simulink model "CM13_2024a_MachE_for_UA_HIL"  (R2024a)
settings: Solver=ode1  StartTime=0.0  StopTime=Inf  FixedStep=0.001  RelTol=1e-3  EnableMultiTasking=on
PreLoadFcn:
  | % if ~length(which('cmcmd')), cmenv; end
PostLoadFcn:
  | if any(exist('dsrtsu_mdlpostloadfcn', 'file') ~= 0), dsrtsu_mdlpostloadfcn('Execute', bdroot); end
InitFcn:
  | , if any(exist('rtifpga_mdlclblib', 'file') ~= 0), rtifpga_mdlclblib('Init', bdroot); end,
  | , if any(exist('dsmpb_private', 'file') ~= 0), dsmpb_private('dsmpb_mdlclblib', 'Init', bdroot); end,
values from neighbouring files (symbols this model uses):
  CoastDown =     [Run_Simulink.mat]
  limitedMCT =     [Run_Simulink.mat]
  MCT =     [Run_Simulink.mat]
  pMCT =     [Run_Simulink.mat]
  RealSimPara =     [Run_Simulink.mat]
  Ref_speed = [13 13.007895099 13.015778396 13.023649891 13.031509584 13.039357475 13.047193564 13.055017851 13.062830336 13.070631019 13.0784199 13.086196979 ... (2669 elements, 2669x1)]    [Ref_speed_and_time.mat]
  Ref_time = [0 0.01 0.02 0.03 0.04 0.05 0.06 0.07 0.08 0.09 0.1 0.11 ... (2669 elements, 2669x1)]    [Ref_speed_and_time.mat]
  US06 =     [Run_Simulink.mat]
undefined symbols (not defined in the file or in its folder): AccelCmd, ActTqLF_Nm_, ActTqLR_Nm_, ActTqRF_Nm_, ActTqRR_Nm_, BattChargeLimitMaxPwr, BattChargeLimitSocBpts, BattChargeLimitTbl, BattChrgCapcty, BattDischargeLimitSocBpts, BattDischargeLimitTbl, BattDischargeMaxPwr, BattNumCellsParallel, BattNumCellsSeries, BattOpenVoltCapBpts, BattOpenVoltTbl, BattResistSocBpts, BattResistTbl, BattResistTempBpts, BrakeMaxPrs, BrakeMaxTrq, ChassisDistCg2FrontAxle, ChassisDistCg2RearAxle, ChassisVehMass, CltchCmd, DecelCmd, DiffRatio, DiscIntNeverNeededParam, EnvGravCnst, EnvPrs, EnvTemp, FuelSpecificGrav, GearCmd, h, InitStates, lgSw, MtrEffSpdBpts, MtrEffTbl, MtrEffTrqBpts, MtrPwrMax, MtrTrqMax, planned_speed, planned_time, ref_speed, ref_time, rticanmm_blockfcn, rticanmm_initfcn, SteeringCmd, SupvsryCtrlRegenBrkCutOffTbl, SupvsryCtrlRegenSpdBpts, TestScnrioCycleNum, VEH
libraries: simulink x264, VSIGenLib x262, etargetslib x201, dsmpblib x161, CarMaker4SL x142, rtimmsu_dsrtlib x32, vehdynlibtire x24, autolibshared x19, vehdynlibsuspension x14, vehdynlibtirecommon x14, autolibutils x10, VsrLibWheel x8
(part 1 of 48)
PreSaveFcn:
  | , if any(exist('dsmpb_private', 'file') ~= 0), dsmpb_private('dsmpb_mdlclblib', 'PreSave', bdroot); end,
CloseFcn:
  | , if any(exist('dsmpb_private', 'file') ~= 0), dsmpb_private('dsmpb_mdlclblib', 'Close', bdroot); end,
settings Model: DataDictionary=DdPassengerEv.sldd  DSMPB_ID_DATA={'10310',struct('BlockId','12f36d3f-3469-493d-9061-ec8dccf8ad98','SignalIds',{{'1d9f63b3-fb1e-42b1-b986-118c3f8e1a5c'}}),'10386',struct('BlockId','00ced8af-8f81-4d96-bdd5-55bcf75b326f','SignalIds',{{'de137f90-4176-4482-a330-2263656912b8','2543f34f-34c7-418b-b364-51a674ed6701','2ea953f6-258f-43af-80b9-296d510766cd','e026f27b-656f-438f-b55c-47d82fb791c0','910672e4-b9cf-495b-ab37-fd8fda6aed4f'}}),'12703',struct('BlockId','d5c239de-9c28-471f-8378-f6be1ca07354','SignalIds',{{'0523bd6f-493f-4b67-9a37-7f171dccadcf'}}),'12768',struct('BlockId','6f08745e-850f-4fc7-99c6-1c2500a944b6','SignalIds',{{'dd9ed340-905e-44be-a84a-808b15caceaf'}}),'12769',struct('BlockId','22e84ecd-9087-47b3-b69e-68ef51f81dd7','SignalIds',{{'a20bbc9a-e0b1-414e-ad46-369f23f85a67'}}),'12770',struct('BlockId','ea678779-fea7-480d-bd70-6fd84e893b88','SignalIds',{{'514a1219-de9e-4b45-a8c1-f0eec9473038'}}),'12849',struct('BlockId','8d70948c-1b65-454e-80b6-488007125876','SignalIds',{{'85315227-9b7c-473a-8f8a-5b34e6a28267'}}),'12850',struct('BlockId','4f95301f-61bc-40f6-b577-b49e4cb81cdc','SignalIds',{{'72592b21-14ea-414f-bad7-eb7b114d5a0e'}}),'12851',struct('BlockId','ac6bf72f-e1b6-495e-9e4b-894c6746d1a0','SignalIds',{{'f9b0dee9-4290-4449-a8ea-24130731cef7'}}),'12857',struct('BlockId','6b10a409-0c93-4934-ac05-3e71bd8b4d56','SignalIds',{{'a7480ea2-3795-4920-80c4-197fbf749da8'}}),'12858',struct('BlockId','c572fa2b-15ad-41aa-81fe-e8bbbed5f461','SignalIds',{{'06004834-c0b9-4189-81f2-9fc7072798a8'}}),'12859',struct('BlockId','1c6655ba-19a9-4cd0-926e-198f5e98e044','SignalIds',{{'527b24a8-f319-412d-b942-e50c619d5c98'}}),'12892',struct('BlockId','cdf75210-031f-4acf-a586-f109f3081db8','SignalIds',{{'0eebc661-386c-4153-975b-200fc7917c9c'}}),'12893',struct('BlockId','bbaf36c3-78c2-4f66-b911-8060317349d0','SignalIds',{{'d6526e73-4ca6-4a7b-95d2-0da9f3f3bb3c'}}),'13389',struct('BlockId','e0063ee2-603a-42f4-80ca-58f4b3e23b5a','SignalIds',{{'5991410c-cc0f-42d8-93ab-94a3aee0e461'}}),'13397',struct('BlockId','0909c5b7-dd88-48d1-abaf-d3324e1e7649','SignalIds',{{'4919af6e-e187-49a8-a288-eb81d671cc8d','e79f3ee3-b422-4636-bed9-529d41626698','8262c110-cc1a-4ba5-8eaa-8176657d5cc1','37cd9612-221b-4281-99cc-4b4394a20fc4','891ab062-363b-41ce-bada-c2e12e4ea74e','cee21b9f-e160-4a13-ad59-480745ef8104','5f399649-cfff-40b7-aace-1cbf0d264993','83711fe8-b2d9-45eb-9dbc-3c51b17f7674','cb7a5443-6e0a-467a-bec9-cb544ca1c2f3'}}),'13398',struct('BlockId','6c3e85bd-363e-417f-8d2b-de29daccd343','SignalIds',{{'573cb497-90a4-454c-b538-934bab3fb65f','4def0a6e-14a7-45d5-ac89-6368950213ca','1faf2666-945f-46a8-b93d-c749f0ec4d9a','255bf974-2f16-4189-ac8d-0135b7b658d1','48de1ef3-4aa0-4b6a-a60f-af052b360edb','b8858909-8a89-4d3a-b884-12439f2c8ddf','7a91e7da-847c-4fed-ac2b-a72166cf88c2','47f03b93-48b4-4b1e-998e-43cb7f69ff32','20de7b31-4a1c-4f17-8b36-e3a815e77dd8'}}),'13399',struct('BlockId','85425dac-ee7a-4bf9-975b-095d7c4dcb51','SignalIds',{{'31f78e19-b7be-40a1-8403-a05f60a9fdd4','54ddbf4f-4a1f-42da-9a57-0479aebd4948','43029009-e5b6-4870-adc7-930fcda97230','fa37dcdd-61b9-427c-8689-e42eb565dcdf','b21329b6-313d-4a80-bafb-48f151b485d6','5e1f092d-d023-45af-8e83-81d7db73fe71','575eb17a-767f-476b-b29e-c7c824fb5c3f'}}),'13400',struct('BlockId','6d25d758-e342-4d0e-a1c0-e299c4d680c4','SignalIds',{{'e44851b8-4536-4fec-815f-e58aadf79b08','786f882c-9ff4-429e-a7c6-066a4a17b40d','45a0b4ca-80fc-40f6-b1e6-27e5d7b713ae','92135807-4645-4e98-a81c-4de8955bda43'}}),'13401',struct('BlockId','9d879170-0616-4207-b220-fd282f7b9eac','SignalIds',{{'ac11617f-dbda-443f-993c-c6fbbd6ab47f','34ee468f-8712-4e56-b2fa-57cfaf4d46a9','6645cccf-1e45-43d8-b9ae-20ca198c39ab','cb498cb6-3450-42a8-8043-9ca37324ef60'}}),'13419',struct('BlockId','43998d1e-e7ec-4013-910a-1b0f7c017215','SignalIds',{{'8d4301fb-cf57-464e-a726-f69194925ee2','74880e10-5ea6-4fdb-851a-33803dc7f46b','6c464908-c4ce-42ec-bd75-49943b5eafb2'}}),'13420',struct('BlockId','e0c48fa1-6a1e-4e4d-a91e-2ca8abf999f7','SignalIds',{{'607599af-e337-41d8-9854-a4c9e0dad2db'}}),'13596',struct('BlockId','2654cd16-1152-433b-ac1a-0269a27feef5','SignalIds',{{'f18cf10c-063a-4024-9056-7b6eead01ef8'}}),'13597',struct('BlockId','4fbf4d76-c906-4f09-a2a6-3f44242523b1','SignalIds',{{'ca8c2ef4-b7df-4c3e-96eb-badff8bb811e'}}),'13598',struct('BlockId','64454236-9a5a-47cb-bb03-f5232c93f512','SignalIds',{{'8d05b93c-46cb-4582-bdb0-e3eb534cd12f'}}),'13599',struct('BlockId','56f11289-4ff5-403f-9839-a82d5b54af48','SignalIds',{{'701aa950-68b2-4ec2-a6c8-d52ba2bcd249'}}),'13600',struct('BlockId','1b0cbb7a-7a69-42f5-9c01-3c170bbe0689','SignalIds',{{'b4817d5e-c060-44db-b5d8-db08f2e889fe'}}),'13601',struct('BlockId','d433aed8-57c8-49ee-bc14-5afa6b45083e','SignalIds',{{'b98e298f-f0b2-450f-b551-4d44ae548aeb'}}),'13602',struct('BlockId','74c1e029-d9b4-4c74-ba04-02cb146b3796','SignalIds',{{'2376ff9a-21ba-487c-823a-f7ab79b5155e'}}),'13603',struct('BlockId','b93cc2c6-1b2f-4cdd-9704-427da45e27fa','SignalIds',{{'e0dbe44a-cc69-4581-af9e-328a90ef1812'}}),'13658',struct('BlockId','9b6a6234-f391-402b-b330-759f0b2f72d0','SignalIds',{{'f5fe7a89-d43d-45da-86dd-9843ffe74786','2b32734c-d92c-4dda-80af-1b7131aac85a','66759741-14ac-464f-974d-6dad41e59beb','2edbc071-bd43-46c5-b834-94c1dd327098','9c492387-aa58-4280-9aa7-95e0d8fe3f01'}}),'13705',struct('BlockId','68defd7b-f812-4d52-8a6f-ab6878e61943','SignalIds',{{'4f92870f-0cc2-427d-ae47-c99b1dd6cbba','06b4d400-fc57-44d8-a8bf-2ee416fb1012','3c4d588d-1906-4006-895e-8fe51fefc384','17ee284c-01e4-44e1-bb0a-5d8f70a5896a','26334ad1-9d74-4531-8fa5-fc841244f7b7'}}),'13706',struct('BlockId','a130b25d-d8e8-4208-976d-a8c4ca165afd','SignalIds',{{'552f6f50-3547-418f-870a-1f967936f110','0b37453a-0fe5-4ef2-9e52-b923bd5f02d1'}}),'13708',struct('BlockId','00e457ba-09c7-460a-8fa7-b07e79c909cf','SignalIds',{{'e82db465-0dc5-4428-9d60-01905a71cf23','4ec6b1dd-22b3-4774-a6d4-013670478f6c','0cfd2b7c-eff3-4a40-9c90-09f8ecc43c65','7fb521d2-5b57-4a71-a2ea-6ccd095d0c8d','0190859d-2e3e-4484-8825-99cc894eeb49','d42c3cfc-c223-4053-93a1-8afdb70193a2'}}),'13709',struct('BlockId','8d7eeffa-57e3-4b4f-84b4-4cf68f00cd15','SignalIds',{{'88d51ca8-c776-4b07-b10b-ccd6deed6120','a40c7935-a03c-429a-b8e5-73a50a866f27','336de083-ceaa-4113-b8ce-44c9d005ade5'}}),'13855',struct('BlockId','35cad703-acce-4db5-b1e1-ecf2bb4e8a68','SignalIds',{{'2413f319-8556-4695-8444-c4a35b6cf84b'}}),'13860',struct('BlockId','2eebd351-5d35-4dc4-8238-5f7ff35a1c0f','SignalIds',{{'a476340e-b09d-48f6-95b7-2a6d936a9864'}}),'13862',struct('BlockId','4cef6eab-d55f-4319-80e1-8f29e1b6ca28','SignalIds',{{'2e3a24d0-c0d4-45f2-b3c3-1f40fcbb9025'}}),'14002',struct('BlockId','b7b542e5-4f26-43e0-af00-0765c47a7be4','SignalIds',{{'b43777bc-78e7-420d-b9c7-924ec3bc0020','d77c6156-a416-4862-952d-fd0c5f3a4268','166ad4cd-0ca0-426d-ae27-28c6d47f4290','eab723f9-c9cb-4bd9-ad26-d5cc16da50d8','51d6cafe-d61a-4ece-aa88-83317d4387c0'}}),'14003',struct('BlockId','690bdae9-44d4-406d-99dc-0fe1eca8290a','SignalIds',{{'6c80bdc4-ebd8-45a9-864d-b0c96184911a','403fc45c-435b-48b1-828c-9b32406d4289'}}),'14004',struct('BlockId','13d1cad0-5e25-434f-942f-03b54b407f13','SignalIds',{{'b6797402-dc17-4702-af16-93cfc7bfd2c6'}}),'14017',struct('BlockId','3f4708ba-c9ff-47b1-b444-ebd911931fcd','SignalIds',{{'60f0e601-d4a2-413a-9877-bf51a75436d8','e9d10586-6241-4149-aed5-74580bd4b32f'}}),'14484',struct('BlockId','7a1b6b1f-e57f-4ef6-b9b6-c00e3a7c18b3','SignalIds',{{'c517a655-c3ae-4248-84d8-a509b79721e3'}}),'14560',struct('BlockId','4b6a7fa7-390d-4c9d-8eb2-f646fefb0631','SignalIds',{{'fda74313-f654-4561-8d6e-e1fa65ef5a21','7ffdead9-2939-42b4-83d3-0e6b32034344','3ef057b8-b6cd-4be8-aee9-398cd49c464f','b4dbcd46-e281-4bb0-843c-cd41170e779c','23ad03d5-e7b7-4ede-a329-18094eaa1732'}}),'14675',struct('BlockId','80315e53-3825-452f-8418-928ce0a5b884','SignalIds',{{'d205fa42-dbb1-4ac4-89fc-174df3da1ad3','8ace96e5-9ccd-4bb6-b3ad-795b8a7818d7'}}),'14676',struct('BlockId','c2ff3260-6d21-42bd-9c67-af339cb9da94','SignalIds',{{'cb4212e4-9c41-4702-928f-e6f7011d53eb','a2441cfe-efec-4f72-80a9-ff18d8aeaeb2'}}),'14677',struct('BlockId','5c259738-61c1-4940-b8c6-678009d700b4','SignalIds',{{'3eaa4d46-076b-4376-8fff-6799fc59ae2c'}}),'14678',struct('BlockId','2b7fdaf0-3bca-4cf8-a01f-16a5ffc40654','SignalIds',{{'7e7316db-c453-4c12-b989-f13ac322e4cc','3324bf27-85f1-4009-b151-35eff7706011'}}),'14748',struct('BlockId','af115fdf-462b-4d46-b5ae-ed48f32a80ce','SignalIds',{{'a2fc24b4-9495-448c-9d68-ee1fbf037ff0','a32c49c5-1f60-4290-a235-9c5ab953ac1f','fbd442c5-8d0d-402d-8b0e-47648da22c93','0dcdade1-2f6f-46b2-a175-bd0a95998b17','aa75d810-8c00-47ac-838d-94ccc8794fde'}}),'14749',struct('BlockId','5bef166d-4a50-45b6-bcd8-c40106e5818d','SignalIds',{{'f4d1b59c-cbd2-4fb4-aba8-393dcc75f58c','0b8133cd-cc0b-4ae3-902f-0805f41a78a0','50798339-b4d9-4001-9b38-71cae5aae466','652cb478-e44a-4f29-9fdc-11278afe8acd','6db05899-163c-4272-b68d-3f23fdc3c2f4'}}),'14863',struct('BlockId','4bdde38d-9bde-4f01-846b-8d6f64c11475','SignalIds',{{'13759f7c-dc26-41c0-a673-d7e6ba4117c6'}}),'14890',struct('BlockId','000dd422-5c9e-49e2-8ae1-d8578451c04f','SignalIds',{{'dd524eb7-1453-448b-a121-3fbe1baeb907','19b407c4-6367-4a79-849c-0e74e550025c','d7d7cf32-1390-4596-8ad8-a7aa1ee97e47','ec108f91-b7ef-4da9-af1a-6887c10d8753'}}),'14895',struct('BlockId','e0a324a1-9c85-4c4d-9120-42a0e22c223f','SignalIds',{{'b3d2bbe9-e87c-45ea-bcce-28bf589283a0','cc171703-e72c-488f-98b6-b3675eb74135','f695ec14-797c-4600-923d-3f8ecde3a7b7'}}),'14908',struct('BlockId','2adb24e4-0efe-45b2-9f22-8475825d43f7','SignalIds',{{'3ceca581-e09a-490b-858b-383b4ff560e2','8daa67bb-bba5-42a9-9ff7-1f642b97bd96'}}),'14916',struct('BlockId','65eb0149-4723-49de-a5d3-69f9fc2610cc','SignalIds',{{'f164dca4-ea5e-462e-b4f1-9f1df6910adb','193413f2-adb8-4371-a123-e7aee3d7ab7f'}}),'15031',struct('BlockId','1f1e6500-410f-49b1-8066-fea9c1ff0cda','SignalIds',{{'ec87fc4e-5b14-4747-9c72-d1e77db60252'}}),'15032',struct('BlockId','6c14e7ad-b236-4cbc-987f-2777f585868c','SignalIds',{{'907d72f5-7c34-4dc8-b661-c51071fe02dc'}}),'15033',struct('BlockId','a2c50340-e125-491b-b6fe-9bd004392e2b','SignalIds',{{'99772446-b668-4d45-9a17-77a327a28077','34fc074f-911c-415d-abca-7890622cc05f'}}),'15034',struct('BlockId','f40daa0e-2494-4582-b47b-fa6e80cc9a9b','SignalIds',{{'904ebebf-fd02-4665-ad45-ede3e402e544','9437c417-61c8-4fd3-8798-da1d3fa95319','fd5d1af9-42ef-4ee3-b09d-926de420ed93','548a470a-bf47-498a-a60e-e5e352f2143e'}}),'15035',struct('BlockId','f52398c5-79fc-42b0-a409-ec3938884e6a','SignalIds',{{'b30d349e-d6a0-44e0-a327-584adaaa49d9'}}),'15036',struct('BlockId','52a4dbb2-6d8c-462d-96a6-dfd44641d89f','SignalIds',{{'289d42f8-ed6e-4801-97a2-d0bf259ebab1','691872a8-7380-4677-9e6c-faf9246f9b43','e0932303-f76d-4dd2-85bc-028033373e8c'}}),'15037',struct('BlockId','0e0291c9-35a5-4563-a570-cb376424caa3','SignalIds',{{'b066e553-674a-4235-9b1a-1f56165c7d67'}}),'2270',struct('BlockId','3bd45aea-114e-4e0b-8274-661c86aceb33','SignalIds',{{'c8b7fc0a-a8e0-4d2f-8a1a-d6be83cb4224'}}),'2773',struct('BlockId','2aba53d9-4d19-4b4d-8397-819e1325edd4','SignalIds',{{'5b2c7b7e-348d-491d-bca0-371c7d75daf6'}}),'2849',struct('BlockId','f460e1ab-e71c-4464-aa19-00052b52454f','SignalIds',{{'30b32590-3625-4bb9-ae32-15e6284ff4a4','66da3457-bf16-43a8-8d28-731e6b8caf4a','952c0afe-8835-4b70-b79b-fdafd7d110e9','fc1acb7d-e31a-4377-87b6-ab40ebaf385e','ba74fcbd-4265-4b9a-9e5b-7274eedbbc92'}}),'3443',struct('BlockId','bf4848e9-a005-4ea5-822a-546d14facefb','SignalIds',{{'59813826-0850-4d64-8d90-ce02e5c4772d'}}),'3444',struct('BlockId','661dc0ac-bd0b-40f3-8260-966d3389d24d','SignalIds',{{'5bd69b46-b717-4764-8a4c-31062ca41d6c'}}),'3445',struct('BlockId','1e60593e-fb4e-4ad7-b476-f227a587c97e','SignalIds',{{'46a8325f-67fa-40bb-92c0-5fbd7b9fd8c0'}}),'3446',struct('BlockId','cf726b69-21f9-4634-b1ea-2afedf885ef4','SignalIds',{{'43cd743a-0c41-42be-aa5c-12364b2a34b1'}}),'3447',struct('BlockId','825c9d59-301a-41c7-ad59-05beda97f4c0','SignalIds',{{'1e421ba1-785f-4677-bc54-4b32ccffbda9'}}),'3448',struct('BlockId','6d4532c8-7821-4780-900f-08e025780dbb','SignalIds',{{'fd5bdd2e-ab61-412d-8d45-c0b4d87df8e1'}}),'3449',struct('BlockId','41cc231b-b267-49ab-a469-ecc9f97ba82b','SignalIds',{{'518b8c22-f5d9-42d6-b2fb-633612b3457c'}}),'3450',struct('BlockId','06ddf642-c8ec-424a-a257-45d7d14fbc9c','SignalIds',{{'191bc148-b179-491d-9c31-5c50bd08bc6c'}}),'3570',struct('BlockId','b840981a-3739-4217-ad3e-20af8bf4bb2c','SignalIds',{{'85ff8f48-ed7c-4597-8ae2-1f0d11eaa759'}}),'3571',struct('BlockId','b44c9645-0f3c-4062-b7ea-542130e6b9d2','SignalIds',{{'0ce735d0-6ea1-4243-b07a-fb60e0271719'}}),'3572',struct('BlockId','a8420ce8-9668-411f-94bd-e6da040620a4','SignalIds',{{'a2d69c3d-b01f-4b76-ba89-e2cf06da7db2'}}),'3648',struct('BlockId','0f5c264c-ffce-4912-adaa-a76aa10f5c95','SignalIds',{{'97ac99fa-5070-4e14-b3c4-316cb4960b65'}}),'3649',struct('BlockId','96f45e98-66f7-475c-982f-1d996f097844','SignalIds',{{'c9d1fa6d-224f-4782-b6fa-e02890b2d4d6'}}),'3650',struct('BlockId','e6f5ddfe-bc8f-44ab-9711-b56df51aee9e','SignalIds',{{'152cb444-4e9c-4a5a-a35b-04356aab4aa1'}}),'3656',struct('BlockId','548c7893-6eac-4873-a730-0dbe400694d8','SignalIds',{{'aed0196a-9e2d-4895-aa85-c8c81f784756'}}),'3657',struct('BlockId','6b692eed-3617-4adc-a523-e5d1ef66fefe','SignalIds',{{'92296544-a098-415a-aa5f-75c942b4cbed'}}),'3658',struct('BlockId','c3916ff6-39b4-422e-aac1-4d4a7e0af62c','SignalIds',{{'7d662d18-9ff5-4e89-b916-88d69295e188'}}),'3738',struct('BlockId','24c81f19-ed3f-4f43-8e7c-e6489392a6df','SignalIds',{{'de091b36-0771-4057-8def-13bdc4ea5265'}}),'3765',struct('BlockId','c267f4c0-5dea-4501-b10d-b1f3fd1bab70','SignalIds',{{'7e394da2-e75e-4490-9c5d-1822b2e5143e','352f2db2-e378-493b-85fb-2e8fa202457f','cd8dd211-ea81-4875-aac8-8e2dcb47c3e2','e1626839-2f5e-4e74-892c-ae50640ccd4b'}}),'3770',struct('BlockId','0b92c14b-9c1e-44ed-9fdf-522f83f38d39','SignalIds',{{'a6b988fe-26fc-4e12-b5c8-bec22bcb8ac3','7587cd01-78be-44f3-94ad-d5cdaef89f1f','9098a390-037c-49bf-addd-6abb7a5009cd'}}),'3783',struct('BlockId','0e03ea55-0f88-465a-82f3-07c0c55c23a2','SignalIds',{{'d79cfbf9-3eee-42b7-83fe-5ffa59395bb0','ecb26389-60a7-4388-bcd5-c3d076c7daa5'}}),'3791',struct('BlockId','5511d4bf-ec34-4089-bd0a-4d2fa1d50221','SignalIds',{{'6e891b67-c300-40f1-9cbe-7c99719c3dea','8e2277c7-98ff-4850-a53a-cbf48bfcf637'}}),'3945',struct('BlockId','RTICANMMMachE_FD1','SignalIds',{{'RTICANMMMachE_FD1'}}),'3946',struct('BlockId','RTICANMMMachE_HS1','SignalIds',{{'RTICANMMMachE_HS1'}}),'3947',struct('BlockId','RTICANMMRCM_ECU','SignalIds',{{'RTICANMMRCM_ECU'}}),'3948',struct('BlockId','RTICANMMRCM_Harness','SignalIds',{{'RTICANMMRCM_Harness'}}),'3987',struct('BlockId','e268d2ed-6e39-4962-b74b-3697adbf2538','SignalIds',{{'9d9d1214-0e83-46e3-82a8-bf2437337278','f2e2d11d-add3-46ca-8702-621238354782','832ad2a4-a12a-4d20-a05f-8b2931d817fe','2b8b2ccb-1185-4cdd-ae35-7cd4304a5dc6','18349be2-9769-4ba0-a538-daf212dea344'}}),'4042',struct('BlockId','3d2d7d32-e11c-44fb-9c6f-d320e9582d7e','SignalIds',{{'70632226-334e-4558-8785-512f47f6587d'}}),'4083',struct('BlockId','8197067e-5b55-4654-bf3a-7d3838659a1e','SignalIds',{{'9f804a3c-ece5-4a4b-bd04-64aaf13b95eb','45cce365-1497-40c9-aa84-16af1661e926','d1caa962-89c6-40e0-a3d7-861511e98cc4','11c79b11-c34d-4913-8abb-889433081684','f5742c5d-3d2a-4fa6-9ac0-daad3352c608','6877a898-e90c-40b9-951f-104101519164','454118bc-a6fa-42b7-82cd-dcbf82ef10ce','951650ed-e53b-4dd3-b6d7-4c5b1fb436a1','a983ea0d-f043-4f0a-ba3f-03e601dd28cb'}}),'4084',struct('BlockId','53121c26-e924-48e8-a1dc-0325cf713f95','SignalIds',{{'324f7103-3f89-420d-bf13-9a25911161ca','90d2717d-392d-4be7-a105-e32120ddcb97','73e292dc-a027-4e20-bea0-5c7f7a52aac6','f84d8076-77c0-4400-9781-46247a4f228c','e88e544c-c1f5-4dab-99fb-16fd9b46c365','f760f4c3-d792-42d1-8cd7-0d38687770ab','344d4755-dfc9-4d1c-845b-a775ec8fb4a2'}}),'4085',struct('BlockId','0a6d60f5-e1ec-4c6e-813b-199248c5f05c','SignalIds',{{'a8b98a70-dea4-4c11-bb6e-857419cf4788','316cba1b-41cb-42dd-8943-bc18f7ffda4c','91169604-1e2f-48a8-9a55-1616419f256f','211cb37d-b04b-4d96-bfc1-0ac855195c7c'}}),'4086',struct('BlockId','554d2636-916a-491c-b89c-72e12efac630','SignalIds',{{'306ecc1d-bc46-4faf-8d20-efaa503ac676','bbaa12f4-bf0e-4ed6-a66f-da9e8c3b5040','288e88f6-b05e-4538-a13b-a1cb6f759554','c458ef25-6454-41c3-8441-d9becbf4dc18','77f978fb-f14e-4abf-b383-5f56beb0de73','7233abf4-5ceb-4740-8c69-db90fa1606e8','1bffef40-6565-4430-8d61-ca520ceacbe4','c3ddf92e-1a7d-4d6f-835a-76d34a4e1e86','80eeb4c2-4c3b-46d1-a845-9d7b6fce451f'}}),'4087',struct('BlockId','9b4880a3-8e4d-4e70-ba55-68100db81fd2','SignalIds',{{'ac7d0d7b-00bb-48d9-b664-32ab2ce281ca','b2b27f5e-8f6f-4fe3-8ce6-155f132e3372','cc0df7e9-940b-496d-9ac8-5b9fcc0aadf2','35a57962-9a8a-46b3-b6f2-3dd4e193c2c9'}}),'4088',struct('BlockId','9701221d-e536-460f-b6ff-ae7caf33fa1a','SignalIds',{{'324f1884-2a22-4f0e-8d5b-fac794e1e49e','1a801da8-464b-48de-986b-4410d9bb9faf','2fa590c2-efe1-4d3e-9e77-b04b5e1964f7'}}),'4141',struct('BlockId','10ebed3e-a81b-4c2d-8bf8-8a780e190cf3','SignalIds',{{'47572e28-138d-4135-b9d8-ccb70b4cc89d','ebee3f8c-ebdb-4ab9-8b8f-d2f779b6e360','4fd8eade-4875-4524-9752-b9d504c58e5d'}}),'4156',struct('BlockId','a9860b6f-1f87-404e-8686-a906221b20ca','SignalIds',{{'95258374-e95d-4ad9-94d8-de012d5dc68a','a5933333-c54b-4ea0-9775-01a673cc1777','f86ce8a3-3c6a-49d0-8a7b-fab6dfe53cf0','eed53fad-0c80-4060-baad-beb21c22aeff','fdcd1b39-5e86-48dd-acd6-694c2f56afe0'}}),'4158',struct('BlockId','0484a6d1-a451-4aee-8580-0e5f289fc0f1','SignalIds',{{'25a1a62f-d854-4a18-b408-79bb5edd6802','2ef09320-d133-41f0-87b8-65fc182e1909','f288fdad-094d-45db-b6a2-7de2a00426ff','79805f85-6d90-40d8-9ab2-0d63d32a2371','8f654a3f-8306-4500-9f0c-b15f6354258e','f0f08236-15cf-4488-aed3-427211bca80d'}}),'4254',struct('BlockId','395a4ea8-d754-45b5-88ed-4fd414dbbaa5','SignalIds',{{'7c79988d-5a47-4b9f-8526-cedc09b18f36','13a3d0cc-0983-401c-bef9-ea241b6b23ab','6671c771-bb09-416e-a09a-694bd8407fd7','171df2ff-ea4d-46ff-99aa-f17cc4a0147f','517a1f0e-b61e-4703-b0b4-6a11c2f9d04f'}}),'4255',struct('BlockId','8f79eb37-105d-4f39-a634-7579a45d6e46','SignalIds',{{'b28aafe4-8cab-4d41-9d2d-2401ff7c522a','653bf2fc-1ac6-48f1-b67a-b81e9f9af1b6'}}),'4257',struct('BlockId','040c599d-8c68-457b-9e1d-e399e302b400','SignalIds',{{'41130444-3422-4cdb-b578-8ddd992cb85d'}}),'4327',struct('BlockId','8481cdf8-4582-4e0f-a3c0-031b81138431','SignalIds',{{'38fc9557-1bd0-481e-823e-14178335dbb3','9f781cac-39af-4702-a354-97d2139a320e','c25fcd5a-5612-4828-816f-ab7904162ef2','1d24290e-5802-431e-a014-bd625f6f5563','ba1dcdfb-2dbd-489d-980a-a99d9489ed3d'}}),'4328',struct('BlockId','11f7f92f-82aa-4e14-8e18-6d45f9f88bbe','SignalIds',{{'a9c38be2-5376-4d0c-a099-f5d5deb160c7','6b863d55-5e81-4068-a020-dff18b0998f9'}}),'4329',struct('BlockId','160e7502-e629-45b2-a9e4-54eada2f4c11','SignalIds',{{'38acdeb5-17e1-49e6-896f-be92b88f5c51','48bcd3d2-64f7-46bd-b241-5da4d93db792'}}),'4349',struct('BlockId','8105b948-2c39-4dc1-b8ce-da8b96ee5c36','SignalIds',{{'437b5a6e-7a7e-4303-950e-e4e47fce2dc6'}}),'4350',struct('BlockId','0d818f62-9726-4d30-90fb-9df933b62db9','SignalIds',{{'b06d9d67-ab30-45a2-a6a1-6548b6f0e336','b94bd36a-2db3-4070-bec6-b9b969879946','670392cd-adeb-40b8-aa81-bd750d435316','ce85f46c-7a8b-4875-8554-5df76678e756','551b3bc8-b2c2-43b5-aeb6-0ca3f4f4d519'}}),'4352',struct('BlockId','ed725d9a-75c7-4890-ad14-af4ea2c6face','SignalIds',{{'3c07e2ab-be23-4ff9-983d-85029b6e5f25'}}),'4353',struct('BlockId','2661ce5a-148d-48ae-9797-9114c14ad1af','SignalIds',{{'7d0705b1-08a9-4b2a-9500-6ec7fbd2b788'}}),'4370',struct('BlockId','ef3b2766-0dbd-48e0-9bfe-80922b4612f6','SignalIds',{{'6d268d3a-d29b-42e9-b488-c4c311ef51c6','214f4fea-3803-4501-9245-acd5cc07d433','bdb283aa-2a53-48cf-8e85-8924aaeeba0f','5d525c66-1f02-49ae-927f-13b892562ddf','ed707b2c-0c09-4ae9-b707-effe353292c9','7b0578b0-4d35-4550-9e9e-2addbe6bfe8c','f545571a-657f-4811-94ad-fe356a840512','44d91631-d9e2-41e9-a43c-452fa71c3e3c','2fe37c30-2ef1-4a80-8047-0f2824863ba7','8dc7ccf1-cf13-4b50-8ef2-ef87533af846','38ce9965-ed63-4361-a37e-b0623d5d3938'}}),'4372',struct('BlockId','05a8bcf8-173d-4a43-b147-b83f4af037f9','SignalIds',{{'b3b22d2c-2c9f-4e4c-832e-a2569b3aedf8','8948ebc4-0f97-4e21-99a6-e029c3794fa9'}}),'4373',struct('BlockId','ddf6f881-a920-4b56-ba4e-b67b7e41a7c8','SignalIds',{{'0255d325-ca08-48fd-a447-e618fd89f68a','a70076de-b40f-41a7-9558-ed3a6b00dbcb'}}),'4696',struct('BlockId','87f299d9-9d53-44c8-8ffa-e55ab40c6501','SignalIds',{{'3707d882-ad49-4c79-bb7b-5b78df9c0f4a'}}),'4718',struct('BlockId','608bab43-b7bd-4ff6-8bec-a00de7ee8ed8','SignalIds',{{'0a71cc3e-01e0-4691-aebf-5597d0218ab7'}}),'4719',struct('BlockId','4d34fc76-85f1-40c1-984c-7605166373d4','SignalIds',{{'da74637e-eba5-4537-a2ae-b8bc9333fdb6','4e64f7a6-3e61-4eb2-80be-5077cdacb374','761903c4-c8ac-4527-95ae-28ca95dc2d64','fc5e6ba2-3b41-4500-aacb-c9cb6bed3f2b'}}),'4720',struct('BlockId','aafb6b7e-be79-4793-885b-2c0adbb8a5fe','SignalIds',{{'602424ee-767e-4c55-8ba5-29361cc527fc'}}),'4721',struct('BlockId','c26c0c53-c634-42b9-9936-b2beb8f11f5b','SignalIds',{{'e048ab61-403c-4a4e-9b3f-3421f417367e'}}),'4726',struct('BlockId','fc4faa17-290c-44b1-8d34-5ab1ff24afa2','SignalIds',{{'308c87d8-fe05-4735-b828-0603c377c865','600a92af-d7a6-4b20-87b5-a8e7489de95b'}}),'4739',struct('BlockId','576a9280-aa1a-4931-857c-d7fd589540b4','SignalIds',{{'f04063fd-6560-42c1-b871-d8137160a897','6f32db81-84d9-4051-ac47-153c9a05de0d','640ffc11-ee96-494b-8bfe-6995eb00a176'}}),'4849',struct('BlockId','529ab12b-5983-4646-9fa2-20483dbcc863','SignalIds',{{'5813fa54-691d-425c-ad99-b92668ff651c','608cdcaa-7e00-4c05-9aa5-cc04d6ae680e','2eea7bf3-f314-4637-af14-61681f413b7e','e44cccb7-15fc-4a75-bc7b-3af80a63ce5d','8e2b1ada-bd78-4adf-b3e0-1b326599dce7','278dd204-65dc-40f7-a9c5-f172a7fbcd8b','bf1e265c-e0dc-4f13-a3bf-ecf679086771','8a159b51-7b24-474d-894a-77003a1e9caf','b8132bd7-9fc8-47f4-beaf-f412ef1581dc','b529718e-249d-45ee-bb57-ffa1754b7c29','7cdae200-1511-49d2-8ef3-d64db997ce6f','35036791-4692-41d7-a4aa-237f69bd50c0','6352a9f1-8d94-4170-8830-71dfc8e8bb47','7589a6e9-758b-4efc-9b55-fb02b3ec1c18','50e8188b-1ff2-44f7-a5b9-f0cdd429d1df','b5163805-0325-4b3e-a3c4-e3b18c5451aa','7db16a25-87c8-40ae-a6a9-8b2dac0999c5','069b5eae-bff4-4019-a800-e924f18d2c08','918bf8d3-1236-4553-96f4-90aac4b13f3f','74bbcf5c-de07-46bb-b1c4-63538cc8a85a','45d0e048-c137-45b2-85ae-98e1ab923db0','bbfa9ab7-7ba7-457a-ace4-abd8c3169042','80e9a2d4-956d-41c2-bbaa-172b2813d3e4','af68c6ce-8d84-4920-be68-88ab1d717e1d','16c13e0d-73f6-40be-b4c6-b1778b128623','f6169fa2-efc6-4124-8e1b-6bbafd8d6002','9a454cee-a777-489e-961b-6f218dae1a4c','ebbfa71f-5964-4338-b234-d2b39fc08c8e','ce6f52c3-c441-4083-bef5-f50324b01608','586f4c1e-0e13-4b79-ab8c-09d4de9c3fa1','37b096d8-3de4-48b6-999b-80c8af92ec0d','f102bb32-825f-4566-bc7f-5c7c63bdd878','f27e54a8-8b6c-4728-a8e5-1561cd647531','ff95cba6-5c0d-4f98-936d-440457fdfae7','32bae0e0-48c8-4e1f-932e-951d34d91d38','449e32b6-a8a5-46de-8b12-50063267d16b','fc3ad2dc-9150-491c-98dc-deed73b93e43','95add159-e4d1-404a-9654-7892cc975445','eedd3bde-9e2c-4eb6-8e18-25a919fc7091','e1c5e27d-8e66-4c29-9dc8-2f8c107165af','45de4045-ce37-4811-887b-53102e3f3fda','e6b1abaa-f2e3-4203-971d-38c784858882','eb4c5f60-7ff4-4819-8004-fa153c51c6ff','5ba96d80-3fc3-4b37-b4b1-a3f148338813'}}),'5227',struct('BlockId','b42573b8-8fd1-4549-b153-71062d83fb1d','SignalIds',{{'25bfa85e-3e58-48e2-81db-cf8121840476'}}),'5233',struct('BlockId','6ec8f5c6-6403-4f2b-abf2-281b17e42fe0','SignalIds',{{'4b09f744-addc-4db4-a041-1a6b8427abf8','a0e7e8ac-9a43-47b4-b459-f1eb45334e7e','60c2eb3c-bd06-4b72-b19e-4a72c026e7b0','8dff12f3-dccf-497c-bfce-2cef66aefc47'}}),'5240',struct('BlockId','576ba332-c54d-4c80-b799-b1e979ee273b','SignalIds',{{'f8bcf20f-39b3-4faf-b6e1-fd3adc0ca8ab'}}),'5241',struct('BlockId','0e9d8633-d564-41b8-a225-51996dd32953','SignalIds',{{'bc09cfc1-3706-42cf-ab19-607d529d31ce'}}),'5247',struct('BlockId','3df4a137-ebd6-42bc-ade8-16f0511a7224','SignalIds',{{'e518c9e9-cdc0-4669-b117-182bb587f387','aa3d50a3-2a08-4b75-9079-d375463f300c'}}),'5248',struct('BlockId','88bacd87-cad4-47a5-8dbd-01190ca807a8','SignalIds',{{'4fda1b19-a520-40d8-adfb-2c56008b191f','30e5f8f7-a6f6-428b-b2a6-f6300f7384fb','2c30290b-e5ec-4877-b6b1-253983b2c2a5'}}),'5515',struct('BlockId','3d93a295-52cb-40ca-bda4-2c156c20ffaa','SignalIds',{{'a604adeb-0398-4bd3-9dd2-c4aaff01e62c'}}),'5516',struct('BlockId','dfff2876-7806-4412-908c-222870e91ddf','SignalIds',{{'50fb3db3-0d00-4d41-931e-4ff654553bab'}}),'5517',struct('BlockId','09e3159c-e585-400a-88e8-8999014bf241','SignalIds',{{'9f289d1f-a081-4275-b4c3-4829c60b9d25'}}),'5592',struct('BlockId','c1121180-6d47-4404-a7df-4948bb16b508','SignalIds',{{'ac2b30a5-5973-4c68-9b8d-36d4064f839a'}}),'5593',struct('BlockId','17cb5b6e-a6c1-4175-b84b-e22e58cd1c5e','SignalIds',{{'8a0ae428-675e-4b16-9731-8d5c6cffa6fd'}}),'5594',struct('BlockId','42ed6673-9dfb-49dd-8cc0-a5654e7b337a','SignalIds',{{'f29b8bff-c848-4c8c-9279-eea7e42705cc'}}),'5600',struct('BlockId','c4747481-2c3b-42e5-8738-162ce36331b4','SignalIds',{{'19c5b6f7-da2e-4eac-ada8-ca47235dfa60'}}),'5601',struct('BlockId','0257c0f9-4bee-4cb0-be05-b43c13cb8587','SignalIds',{{'8f6ff0b3-f66d-460c-ad5c-a09b350e3156'}}),'5602',struct('BlockId','c9e19b64-ef7e-4da3-abd2-7665e3db4d9b','SignalIds',{{'90386a0d-cec0-4aec-97a6-07063c2b445c'}}),'5631',struct('BlockId','78774a71-872e-499e-ac80-40eef33bf6d4','SignalIds',{{'0fbc09aa-6fea-4c64-9ba5-60b4f66cb649'}}),'5632',struct('BlockId','b5beacde-0424-4e19-a59b-be18f75db7b1','SignalIds',{{'3a999b22-e93f-46e4-9475-163dbc6052fd'}}),'6168',struct('BlockId','95b8c2d2-f6ae-4e8b-b08b-c1f112b44fde','SignalIds',{{'519a5d69-ed82-4ebd-8eec-63a8e47c1d29'}}),'6176',struct('BlockId','26228621-a802-4aeb-856e-4e4f8da015e8','SignalIds',{{'8715b19a-486c-4fb0-a7ad-778d101cfe5e','ededd69a-f703-458f-a5bc-d5de56e9b231','84fdfcaf-5077-4cd8-adea-505a250c7374','f9346eba-68fe-48f5-b6ae-117ee2e1aa47','5e4d9eb1-05bd-47bd-81ee-c483b45a07e9'}}),'6177',struct('BlockId','4db81051-2445-4a70-a4c4-e85e051221ac','SignalIds',{{'fa2052be-519a-4340-bc28-88af64b4d5af','b26659fc-c0fa-42ce-bb1f-08b44739add2'}}),'6181',struct('BlockId','b7d7f87d-5783-4b40-8512-e8c4728040f1','SignalIds',{{'18bff9ba-963d-4a7e-a634-08045cdeb052'}}),'6671',struct('BlockId','f9872320-fe22-4001-b512-6380e1d4e736','SignalIds',{{'21296f63-1fee-44a6-b133-b8eb5d072cc4'}}),'6747',struct('BlockId','e0d8f2db-cd23-43c8-81d6-d68e66f94990','SignalIds',{{'11390e12-efe1-4fcc-a0ed-13cc8c1dd6ad','ac9e9c38-c41c-4cbf-b724-94ed7006e061','e3f12f3a-8e34-4884-a163-bcb02ccf114e','b07b523d-c8bd-4e60-8b2d-f38ea134d00b','511e7d66-1863-4f40-92c4-b5cc9d9aa8de'}}),'9182',struct('BlockId','d74564a3-d995-4912-b589-32bbe6269602','SignalIds',{{'fb69f55e-8804-409b-b344-5bace57d37dd'}}),'9183',struct('BlockId','72013167-b4b0-42db-9197-3f06e134379c','SignalIds',{{'59ef9486-c48c-4bc9-8b99-fb647c468003'}}),'9184',struct('BlockId','6ec74d48-56e3-4762-8cc8-7b19ff8368ce','SignalIds',{{'30acef2d-06f3-4dfe-8c85-21be6e8447ee'}}),'9259',struct('BlockId','34501448-c21e-4be1-a030-67f37b4e60ea','SignalIds',{{'6d8db6e2-941e-47b5-b56b-d7bb2b92ff2d'}}),'9260',struct('BlockId','4522a02d-00f2-400b-b99b-11796a136b36','SignalIds',{{'04289263-70eb-457f-bfc7-12be2e4f58a5'}}),'9261',struct('BlockId','581a38d9-c008-4c5a-bbda-18f0ef0fb430','SignalIds',{{'5d1f7e4c-ae0c-431c-9770-fe6294a744ef'}}),'9267',struct('BlockId','2e40b220-02e0-4b2b-925b-0cd163ecae7e','SignalIds',{{'5fbe4c33-8653-4e49-9cf4-980a3141e788'}}),'9268',struct('BlockId','c83ca69a-3d0e-4561-9216-1cd5e6b7fc91','SignalIds',{{'ef822cb5-4a67-4824-aec0-8d7404dd07b0'}}),'9269',struct('BlockId','6098b033-afd9-4222-a8bd-e728ee1b6496','SignalIds',{{'e63f90e3-cf21-4301-bb7d-c8b342c71866'}}),'9298',struct('BlockId','72837867-8f2d-4f36-8099-921b89fdc76b','SignalIds',{{'6aed80f0-ded6-4fc8-b3a4-81de4b77f965'}}),'9299',struct('BlockId','e0ba81a7-ee7a-4df7-a52d-57e875caa1d7','SignalIds',{{'6669b16f-a15c-46f4-8ec3-6d1d2ef9e57b'}}),'9807',struct('BlockId','261cb522-9808-4bc1-8122-27e0c7dd6200','SignalIds',{{'acdd3b2a-c7a0-4f7c-b3b3-aa55f7518519'}}),'9815',struct('BlockId','8b60a9f2-f8b4-467f-a001-aef853797dd6','SignalIds',{{'4c0c9a14-e0a1-4674-b31b-877822bd9a81','06703d3d-9d28-4ab2-866b-5deff86fe5bb','d9157d0b-f3d4-435d-8a02-5b4a15e9b192','a8d3d9ab-ad47-452f-bd6b-2c706751ddec','96249f07-2ae6-48e1-b7e2-35fa2c76ed3a'}}),'9816',struct('BlockId','62cbc5e1-477f-40e5-9a52-3c46b63d5ba8','SignalIds',{{'40f8e1c1-a8f0-4a34-b03d-72eb96768064','da2e89e2-9082-4f7e-9d08-8d6bbdf3d7dc'}}),'9820',struct('BlockId','5cca28c4-a169-4a9a-895a-4073fb9a218d','SignalIds',{{'938e091a-2900-4b2f-baa3-47f95ffa096f'}})}  RTICANMMDATA=struct('GeneralSetupData',struct('modelroot','C:\CM_Projects\UA_cave\CM13_proj\src_cm4dspace_realsim','generalsettings',struct('filesettings',struct('destfolder',struct('Name','RTICANMM_FILES','Check',1),'buildfolder',struct('Name','.','Check',1),'AbsDestfolder',struct('Name','C:\CM_Projects\UA_cave\CM13_proj\src_cm4dspace_realsim\RTICANMM_FILES'),'AbsBuildfolder',struct('Name','C:\CM_Projects\UA_cave\CM13_proj\src_cm4dspace_realsim'))),'options',struct('addpaths',1,'rmpaths',1,'addtrcexclusion',true,'cannavigator',struct('checkmonitoring',0),'show_usrtrc',0,'use_usrtrc',0,'addpath2usrmk',1),'advanced',struct('options',ones(1,100)),'MPSetup',{{}},'modelname','CM13_2024a_MachE','blockdata',struct('generalsettings',struct('filesettings',struct('destfolder',struct('Name','.','Check',1),'AbsDestfolder',struct('Name','T:\TOOL_SOURCES\CANnedy\m'),'buildfolder',struct('Name','.','Check',1),'AbsBuildfolder',struct('Name','C:\MATLAB6p5\work'))),'options',struct('addpaths',1,'rmpaths',1,'addpath2usrmk',1),'modelname','rticanmmlib','modelroot','T:\TOOL_SOURCES\CANnedy\m'),'MMType','RTICANMM','block',['CM13_2024a_MachE/CarMaker/IPG Vehicle/MachE CAN/RTICANMM' char(10) 'GeneralSetup'],'RTI',struct('Type','DSRT','Ver','24.1','Date','02-May-2024'),'version','24.1.739338.0305092592','userdata',struct('HostServiceChannelID',{{'MachE_FD1','RCM_ECU','RCM_Harness','MachE_HS1',[]}})))  DSRTSU_INTERNAL_RTIFPGA=210  DSRTSU_INTERNAL_RTISTBM_VER=24.1  Creator=CAVE  LastModifiedBy=RVDP
settings SolverCC: AlgebraicLoopSolver=TrustRegion
settings DataIOCC: LimitDataPoints=on  SaveFormat=Array  SignalLoggingSaveFormat=ModelDataLogs  SignalLogging=off  ReturnWorkspaceOutputs=off  SignalLoggingName=sigsOut
settings OptimizationCC: BlockReduction=off  BooleanDataType=off  ConditionallyExecuteInputs=off  OptimizeBlockIOStorage=off  BufferReuse=off  ExpressionDepthLimit=2147483647  InitFltsAndDblsToZero=on
settings DebuggingCC: SaveWithParameterizedLinksMsg=none  MergeDetectMultiDrivingBlocksExec=none  SignalResolutionControl=TryResolveAllWithWarning  MultiTaskDSMMsg=warning  MultiTaskCondExecSysMsg=none  TasksWithSamePriorityMsg=none  FcnCallInpInsideContextMsg=warning  UnconnectedInputMsg=warning  UnconnectedOutputMsg=warning  UnconnectedLineMsg=warning  StateNameClashWarn=warning  SFUnexpectedBacktrackingDiag=warning  SFNoUnconditionalDefaultTransitionDiag=warning  ArithmeticOperatorsInVariantConditions=warning
settings HardwareCC: ProdBitPerLong=64  ProdLargestAtomicInteger=Integer  ProdWordSize=32  ProdLongLongMode=on  ProdHWDeviceType=Custom Processor->Custom
settings ModelReferenceCC: EnableRefExpFcnMdlSchedulingChecks=on  EnableParallelModelReferenceBuilds=on  PropagateSignalLabelsOutOfModel=off
settings SFSimCC: SimUseLocalCustomCode=off  CustomCodeUndefinedFunction=UseInterfaceOnly
settings RTWCC: Description=dSPACE Target DSRT - Generates SIC files for import by ConfigurationDesk and VEOS. Provides code generation for Simulink models imported in ConfigurationDesk.  SystemTargetFile=dsrt.tlc  GenCodeOnly=on  MakeCommand=make_dsrt  TemplateMakefile=dsrt_default_tmf  RTWVerbose=off  RTWUseLocalCustomCode=off  GPUComputeCapability=3.5  DLArmComputeVersion=19.05
settings CodeAppCC: MaxIdLength=63  StateflowObjectComments=on
settings STFCustomTargetCC: TargetLangStandard=C89/C90 (ANSI)  ParMdlRefBuildCompliant=on  GRTInterface=off  UseToolchainInfoCompliant=off  SystemTargetFile=dsrt.tlc
settings GRTTargetCC: TargetLangStandard=C89/C90 (ANSI)  CompOptLevelCompliant=off  ConcurrentExecutionCompliant=off  CombineOutputUpdateFcns=off  MatFileLogging=off  CPPClassGenCompliant=off  UseToolchainInfoCompliant=off  RTWCAPISignals=on
settings ConfigComp: CovMetricSettings=dw  CovSaveCumulativeToWorkspaceVar=on  CovSaveSingleToWorkspaceVar=on  CovExternalEMLEnable=off

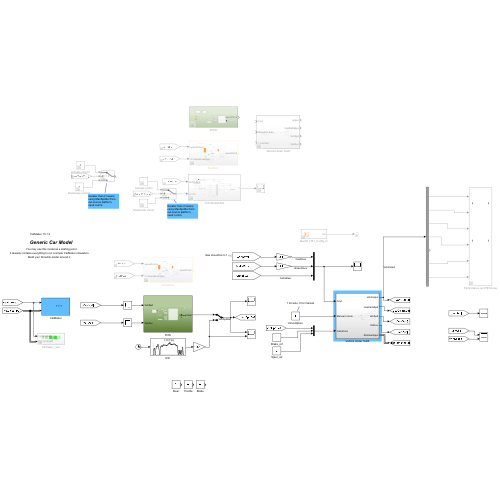
[thumbnail: Simulink's stored preview of the top-level diagram]
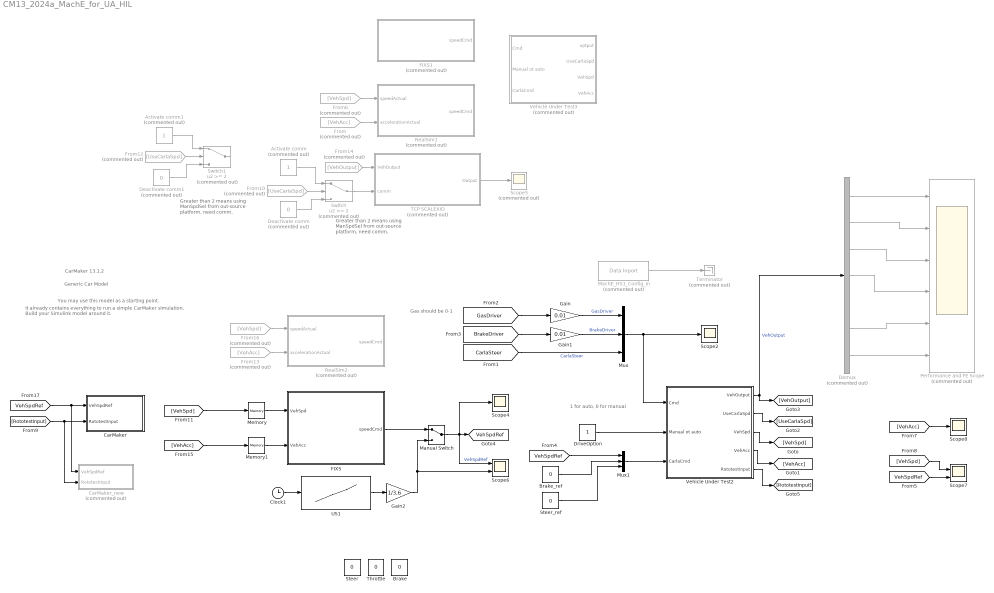
== system CM13_2024a_MachE_for_UA_HIL ==
  note: Generic Car Model
  note: You may use this model as a starting point.
  note: It already contains everything to run a simple CarMaker simulation.
      | Build your Simulink model around it.
  note: CarMaker 13.1.2
  note: Greater than 2 means using ManSpdSel from out-source platform, need comm.
  note: Greater than 2 means using ManSpdSel from out-source platform, need comm.
  note: 1 for auto, 0 for manual
  note: Gas should be 0-1
  Activate comm : Constant  Commented=on
  Activate comm1 : Constant  Commented=on
  Brake : Constant  Value=0
  Brake_ref : Constant  Value=0
  CarMaker : Subsystem
      mask Display: image(imread('CarMakerSys.png'));
  CarMaker_new : Subsystem  Commented=on
  Clock1 : Clock
  Deactivate comm : Constant  Commented=on  Value=0
  Deactivate comm1 : Constant  Commented=on  Value=0
  Demux : Demux  Commented=on  Outputs=7
  DriveOption : Constant
  FIXS : Subsystem
  FIXS1 : Subsystem  Commented=on
  From : From  Commented=on  GotoTag=VehAcc
  From10 : From  Commented=on  GotoTag=UseCarlaSpd
  From12 : From  Commented=on  GotoTag=UseCarlaSpd
  From13 : From  Commented=on  GotoTag=VehAcc
  From14 : From  Commented=on  GotoTag=VehOutput
  From16 : From  Commented=on  GotoTag=VehSpd
  From6 : From  Commented=on  GotoTag=VehSpd
  Gain : Gain  Gain=0.01
  Gain1 : Gain  Gain=0.01
  Gain2 : Gain  Gain=1/3.6
  MachE_HS1_Config_In : dsmpblib/Data Inport  Priority=10000  Commented=on
      settings: SourceProductName=dSPACE Model Interface Package for Simulink (MIPS)
  Manual Switch : ManualSwitch
  Memory : Memory
  Memory1 : Memory
  Mux : Mux  Inputs=3
  Mux1 : Mux  Inputs=3
  Performance and FE Scope : Scope  Commented=on  NumInputPorts=6
  RealSim1 : Subsystem  Commented=on
  RealSim2 : Subsystem  Commented=on
  Scope2 : Scope
  Scope4 : Scope
  Scope5 : Scope  Commented=on
  Scope6 : Scope  NumInputPorts=2
  Scope7 : Scope  NumInputPorts=2
  Scope8 : Scope
  Steer : Constant  Value=0
  Steer_ref : Constant  Value=0
  Switch : Switch  Commented=on  Threshold=2  SaturateOnIntegerOverflow=off  InputSameDT=off
  Switch1 : Switch  Commented=on  Threshold=2  SaturateOnIntegerOverflow=off  InputSameDT=off
  TCP SCALEXIO : Subsystem  Commented=on
  Terminator : Terminator  Commented=on
  Throttle : Constant  Value=0
  US1 : Lookup_n-D  NumberOfTableDimensions=1  BreakpointsForDimension1=US06.Time  Table=US06.Speed  InternalRulePriority=Speed  RndMeth=Simplest
  Vehicle Under Test2 : Subsystem
  Vehicle Under Test3 : Subsystem  Commented=on
  tag scope: VehSpdRef=global
  wires:
  Demux/1 -> Performance and FE Scope/1
  Memory/1 -> FIXS/1(VehSpd)
  Gain/1 -> Mux/1  "GasDriver"
  From13/1 -> RealSim2/2(accelerationActual)
  Demux/2 -> Performance and FE Scope/2
  Demux/6 -> Performance and FE Scope/5
  From16/1 -> RealSim2/1(speedActual)
  [VehSpdRef] -> Scope7/2
  Activate comm/1 -> Switch/1
  Memory1/1 -> FIXS/2(VehAcc)
  Clock1/1 -> US1/1
  [VehSpd] -> Scope7/1
  Vehicle Under Test2/4(VehAcc) -> [VehAcc]
  Deactivate comm1/1 -> Switch1/3
  Activate comm1/1 -> Switch1/1
  Mux/1 -> Vehicle Under Test2/1(Cmd), Scope2/1
  [VehAcc] -> Memory1/1
  Demux/7 -> Performance and FE Scope/6
  Demux/4 -> Performance and FE Scope/4
  Mux1/1 -> Vehicle Under Test2/3(CarlaCmd)
  [VehSpdRef] -> Mux1/1
  Demux/3 -> Performance and FE Scope/3
  From10/1 -> Switch/2
  Vehicle Under Test2/2(UseCarlaSpd) -> [UseCarlaSpd]
  Manual Switch/1 -> Scope4/1, Scope6/1, [VehSpdRef]  "VehSpdRef"
  Steer_ref/1 -> Mux1/3
  From/1 -> RealSim1/2(accelerationActual)
  Brake_ref/1 -> Mux1/2
  DriveOption/1 -> Vehicle Under Test2/2(Manual ot auto)
  From6/1 -> RealSim1/1(speedActual)
  US1/1 -> Gain2/1
  Switch/1 -> TCP SCALEXIO/2(comm)
  [VehAcc] -> Scope8/1
  [CarlaSteer] -> Mux/3  "CarlaSteer"
  Deactivate comm/1 -> Switch/3
  Vehicle Under Test2/3(VehSpd) -> [VehSpd]
  FIXS/1(speedCmd) -> Manual Switch/1
  [GasDriver] -> Gain/1
  [VehSpd] -> Memory/1
  Vehicle Under Test2/1(VehOutput) -> [VehOutput], Demux/1  "VehOutput"
  TCP SCALEXIO/1(Output) -> Scope5/1
  From14/1 -> TCP SCALEXIO/1(VehOutput)
  Gain1/1 -> Mux/2  "BrakeDriver"
  [BrakeDriver] -> Gain1/1
  MachE_HS1_Config_In/1 -> Terminator/1
  Gain2/1 -> Scope6/2, Manual Switch/2
  From12/1 -> Switch1/2
  Vehicle Under Test2/5(RototestInput) -> [RototestInput]
  [VehSpdRef] -> CarMaker/1(VehSpdRef), CarMaker_new/1(VehSpdRef)
  [RototestInput] -> CarMaker/2(RototestInput), CarMaker_new/2(RototestInput)

== system CM13_2024a_MachE_for_UA_HIL/CarMaker ==
  VehSpdRef : Inport
  RototestInput : Inport  Port=2
  CM_FIRST : Subsystem  Commented=on
  CM_LAST : Subsystem  Commented=on
  DrivMan : Subsystem  Commented=on
  Ground : Ground
  IPG Vehicle : Subsystem
  Terminator : Terminator
  VehicleControl : Subsystem
  wires:
  DrivMan/2(DrivMan.Out) -> VehicleControl/2(DrivMan.In)
  DrivMan/1(Sync_Out) -> VehicleControl/1(Sync_In)
  CM_FIRST/2(Env.Misc) -> DrivMan/2(Env.Misc)
  CM_FIRST/1(Sync_Out) -> DrivMan/1(Sync_In)
  CM_LAST/1(Sync_Out) -> Terminator/1
  Ground/1 -> CM_FIRST/1(Sync_In)
  IPG Vehicle/1(Sync_Out) -> CM_LAST/1(Sync_In)
  VehicleControl/1(Sync_Out) -> IPG Vehicle/1(Sync_In)
  VehicleControl/3(VhclCtrl.Steering) -> IPG Vehicle/3(VhclCtrl.Steering)
  VehicleControl/4(Vhcl.Wheel.In) -> IPG Vehicle/4(Vhcl.Wheel.In)
  VehicleControl/5(Vhcl.Misc) -> IPG Vehicle/5(Vhcl.Misc)
  VehicleControl/6(VhclCtrl.Brake) -> IPG Vehicle/6(VhclCtrl.Brake)
  VehicleControl/7(VhclCtrl.PT) -> IPG Vehicle/7(VhclCtrl.PT)
  VehicleControl/2(Vhcl.Model.Source) -> IPG Vehicle/2(Vhcl.Model.Source)
  IPG Vehicle/2(CAVE_Driver) -> VehicleControl/3(CAVE_driver)
  VehSpdRef/1 -> IPG Vehicle/8(VehSpdRef)
  RototestInput/1 -> IPG Vehicle/9(RototestInput)

== system CM13_2024a_MachE_for_UA_HIL/CarMaker_new ==
  VehSpdRef : Inport
  RototestInput : Inport  Port=2
  CM_FIRST : Subsystem  Commented=on
  CM_LAST : Subsystem  Commented=on
  DrivMan : Subsystem  Commented=on
  Ground : Ground
  IPG Vehicle : Subsystem
  Terminator : Terminator
  VehicleControl : Subsystem
  wires:
  VehSpdRef/1 -> IPG Vehicle/8(VehSpdRef)
  Ground/1 -> CM_FIRST/1(Sync_In)
  CM_FIRST/1(Sync_Out) -> DrivMan/1(Sync_In)
  CM_LAST/1(Sync_Out) -> Terminator/1
  CM_FIRST/2(Env.Misc) -> DrivMan/2(Env.Misc)
  DrivMan/1(Sync_Out) -> VehicleControl/1(Sync_In)
  IPG Vehicle/2(CAVE_Driver) -> VehicleControl/3(CAVE_driver)
  RototestInput/1 -> IPG Vehicle/9(RototestInput)
  IPG Vehicle/1(Sync_Out) -> CM_LAST/1(Sync_In)
  VehicleControl/5(Vhcl.Misc) -> IPG Vehicle/5(Vhcl.Misc)
  VehicleControl/6(VhclCtrl.Brake) -> IPG Vehicle/6(VhclCtrl.Brake)
  VehicleControl/7(VhclCtrl.PT) -> IPG Vehicle/7(VhclCtrl.PT)
  VehicleControl/2(Vhcl.Model.Source) -> IPG Vehicle/2(Vhcl.Model.Source)
  DrivMan/2(DrivMan.Out) -> VehicleControl/2(DrivMan.In)
  VehicleControl/4(Vhcl.Wheel.In) -> IPG Vehicle/4(Vhcl.Wheel.In)
  VehicleControl/1(Sync_Out) -> IPG Vehicle/1(Sync_In)
  VehicleControl/3(VhclCtrl.Steering) -> IPG Vehicle/3(VhclCtrl.Steering)

== system CM13_2024a_MachE_for_UA_HIL/FIXS ==
  note: This flag will bypass all other logic and force the ramp down of HIL
  VehSpd : Inport
  VehAcc : Inport  Port=2
  Clock : Clock
  Constant : Constant  Value=RealSimPara.speedInit
  DistanceTravel (m) : Constant  Value=0
  Gain3 : Gain  Gain=3.6
  Manual Switch : ManualSwitch  CurrentSetting=0
  Manual Switch1 : ManualSwitch
  RampDownFlag : Constant  Value=0
  RampUpFlag : Constant  Value=0
  RealSim Core : Subsystem
  RealSimHILCycle : Stateflow chart  TreatAsAtomicUnit=on
  SimState : Constant  Value=10
  SimTime : Constant  Value=10
  Terminator{,1..4} (5 alike) : Terminator
  initialWaitTime : Constant  Value=0
  totalDistance (m) : Constant  Value=1000000
  totalTime (sec) : Constant  Value=10000
  speedCmd : Outport
  wires:
  RealSim Core/2(speedDesiredIn) -> Terminator/1
  RampDownFlag/1 -> RealSimHILCycle/9(RampDownFlag)
  totalDistance (m)/1 -> RealSimHILCycle/7(totalDistance)
  Manual Switch/1 -> RealSimHILCycle/3(SpeedIn)
  Gain3/1 -> Terminator1/1  "HIL_SpeedCmd_kph"
  totalTime (sec)/1 -> RealSimHILCycle/8(totalTime)
  RealSimHILCycle/1(CycleMode) -> Terminator3/1  "CycleMode"
  initialWaitTime/1 -> RealSimHILCycle/5(InitWaitTime)
  RealSimHILCycle/2(SpeedCmd) -> [HIL_SpeedCmd], Manual Switch1/2, Gain3/1
  Constant/1 -> Manual Switch/1, RealSimHILCycle/6(SpeedInit)
  Manual Switch1/1 -> speedCmd/1
  RealSim Core/3(speedCmd) -> Manual Switch1/1, Manual Switch/2
  RampUpFlag/1 -> RealSimHILCycle/10(RampUpFlag)
  VehSpd/1 -> RealSim Core/1(VehSpd)
  RealSim Core/1(VehDataBusIn) -> Terminator2/1
  RealSim Core/4(speedActual) -> Terminator4/1
  DistanceTravel (m)/1 -> RealSimHILCycle/4(DistanceTravel)
  SimState/1 -> RealSimHILCycle/2(SimState)
  Clock/1 -> RealSimHILCycle/1(SimTime)
  VehAcc/1 -> RealSim Core/2(VehAcc)

== system CM13_2024a_MachE_for_UA_HIL/FIXS1 ==
  note: This flag will bypass all other logic and force the ramp down of HIL
  Constant : Constant  Value=RealSimPara.speedInit
  Gain3 : Gain  Gain=3.6
  Manual Switch : ManualSwitch  CurrentSetting=0
  Manual Switch1 : ManualSwitch  CurrentSetting=0
  RampDownFlag : Constant  Value=0
  RampUpFlag : Constant  Value=0
  Read CM Dict3 : CarMaker4SL/Read CM Dict  xname=Time  xsync=off  xstime=Continuous
  Read CM Dict7 : CarMaker4SL/Read CM Dict  xname=SC.State  xsync=off  xstime=Continuous
  Read CM Dict8 : CarMaker4SL/Read CM Dict  xname=Vhcl.Distance  xsync=off  xstime=Continuous
  RealSim Core : Subsystem
  RealSim Translate CM Signal to Bus as Feedback to SUMO/VISSIM : Subsystem
  RealSimHILCycle : Stateflow chart  TreatAsAtomicUnit=on
  Terminator : Terminator
  Terminator1 : Terminator
  Terminator3 : Terminator
  initialWaitTime : Constant  Value=10000
  totalDistance (m) : Constant  Value=1000000
  totalTime (sec) : Constant  Value=10000
  speedCmd : Outport
  wires:
  RealSim Translate CM Signal to Bus as Feedback to SUMO/VISSIM/1(VehDataBusOut) -> RealSim Core/1(VehDataBusOut)
  RealSim Core/2(speedDesiredIn) -> Terminator/1
  RealSim Core/1(VehDataBusIn) -> RealSim Translate CM Signal to Bus as Feedback to SUMO/VISSIM/1(VehDataBusIn)
  RealSim Translate CM Signal to Bus as Feedback to SUMO/VISSIM/2(CM_speed) -> RealSim Core/2(CM_speed)
  RampDownFlag/1 -> RealSimHILCycle/9(RampDownFlag)
  totalDistance (m)/1 -> RealSimHILCycle/7(totalDistance)
  Manual Switch/1 -> RealSimHILCycle/3(SpeedIn)
  Gain3/1 -> Terminator1/1  "HIL_SpeedCmd_kph"
  totalTime (sec)/1 -> RealSimHILCycle/8(totalTime)
  RealSimHILCycle/1(CycleMode) -> Terminator3/1  "CycleMode"
  initialWaitTime/1 -> RealSimHILCycle/5(InitWaitTime)
  RealSimHILCycle/2(SpeedCmd) -> [HIL_SpeedCmd], Manual Switch1/2, Gain3/1
  Constant/1 -> RealSimHILCycle/6(SpeedInit), Manual Switch/1
  [DistanceTravel] -> RealSimHILCycle/4(DistanceTravel)
  [SimState] -> RealSimHILCycle/2(SimState)
  [CM_Time] -> RealSimHILCycle/1(SimTime)
  Manual Switch1/1 -> speedCmd/1
  RealSim Core/3(speedCmd) -> Manual Switch/2, Manual Switch1/1
  Read CM Dict7/1 -> [SimState]  "SimCore_State"
  Read CM Dict8/1 -> [DistanceTravel]  "distanceTravel"
  Read CM Dict3/1 -> [CM_Time]  "CM_Time"
  RampUpFlag/1 -> RealSimHILCycle/10(RampUpFlag)
  RealSim Core/4(speedActual) -> RealSim Translate CM Signal to Bus as Feedback to SUMO/VISSIM/2(speedActual)
